simulink model "misura_PI_D"  (R2017a)
settings: Solver=VariableStepAuto  StartTime=0.0  StopTime=2000  RelTol=1e-3
values from neighbouring files (symbols this model uses):
  kP = 1.2684    [PI.m]    (also in PID.m = 1; PI_D.m = 1)
  N = 5    [margine_fase.m]    (also in stima_grafica_I_ordine.m = 30)
  Ti = 1    [PID.m]    (also in PI_D.m)
undefined symbols (not defined in the file or in its folder): Td
libraries: cstblocks x1
settings Model: Creator=Enrico Donato  LastModifiedBy=Enrico Donato

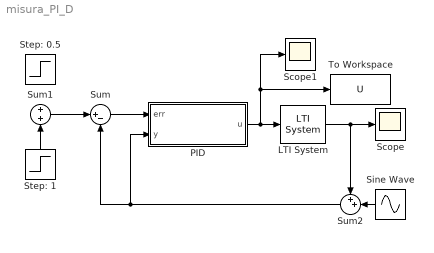
== system misura_PI_D ==
  LTI System : cstblocks/LTI System  sys=G  IC=[]
  "PID " : Subsystem
  Scope : Scope
  Scope1 : Scope
  Sine Wave : Sin  Amplitude=1/1000  Frequency=100  SampleTime=0
  Step: 0.5 : Step  Time=10  After=0.5  SampleTime=0
  Step: 1 : Step  Time=0  SampleTime=0
  Sum : Sum  Inputs=|+-
  Sum1 : Sum  Inputs=+|+
  Sum2 : Sum  Inputs=++|
  To Workspace : ToWorkspace  VariableName=U  SaveFormat=Timeseries  SampleTime=-1
  wires:
  "PID "/1(u) -> LTI System/1, To Workspace/1, Scope1/1
  Sum/1 -> "PID "/1(err)
  LTI System/1 -> Sum2/1, Scope/1
  Sum1/1 -> Sum/1
  Step: 1/1 -> Sum1/2
  Sine Wave/1 -> Sum2/2
  Sum2/1 -> "PID "/2("y "), Sum/2

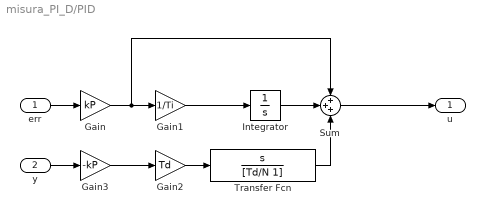
== system misura_PI_D/PID  ==
  err : Inport
  "y " : Inport  Port=2
  Gain : Gain  Gain=kP
  Gain1 : Gain  Gain=1/Ti
  Gain2 : Gain  Gain=Td
  Gain3 : Gain  Gain=-kP
  Integrator : Integrator
  Sum : Sum  Inputs=+++
  Transfer Fcn : TransferFcn  Numerator=[1 0]  Denominator=[Td/N 1]
  u : Outport
  wires:
  Sum/1 -> u/1
  err/1 -> Gain/1
  Gain1/1 -> Integrator/1
  Integrator/1 -> Sum/2
  Gain/1 -> Gain1/1, Sum/1
  Gain2/1 -> Transfer Fcn/1
  Gain3/1 -> Gain2/1
  "y "/1 -> Gain3/1
  Transfer Fcn/1 -> Sum/3
